simulink model "sensor_fusion"  (R2026a)
settings: Solver=ode1  StopTime=Inf  FixedStep=1/60
PostLoadFcn:
  | qlabs_setup
model workspace (MAT data in the model file):
  lidarStepSize = 0.2
  mainStepSize = Simulink.Parameter
  mainStepSize.Value = Simulink.data.Expression
  mainStepSize.Value.ExpressionString = "qc_get_step_size"
  mainStepSize.Complexity = 'real'
  mainStepSize.Dimensions = -1
  mainStepSize.DataType = 'auto'
  mode = Simulink.Parameter
  mode.Value = 1
  mode.Complexity = 'real'
  mode.Dimensions = [1 1]
  mode.Description = '0 - education speeds via wheel speed commands
    | 1 - education speeds via body speed commands
    | 2 - research speeds via wheel speed commands
    | 3 - research speeds via body speed commands'
  mode.DataType = 'auto'
  realSenseStepSize = Simulink.Parameter
  realSenseStepSize.Value = Simulink.data.Expression
  realSenseStepSize.Value.ExpressionString = "qc_get_step_size*ceil(1/30/qc_get_step_size)"
  realSenseStepSize.Complexity = 'real'
  realSenseStepSize.Dimensions = -1
  realSenseStepSize.DataType = 'auto'
undefined symbols (not defined in the file or in its folder): Point
libraries: quarc_library x17, simulink x1
settings Model: ExtModeTrigDuration=10000  Creator=mbohra  LastModifiedBy=rdu
settings DebuggingCC: UnderspecifiedInitializationDetection=Classic
settings SimscapeCC: SimscapeNominalValues="[{\"value\":\"1\",\"unit\":\"A\"},{\"value\":\"1\",\"unit\":\"bar\"},{\"value\":\"1\",\"unit\":\"cm^2\"},{\"value\":\"1\",\"unit\":\"cm^3/s\"},{\"value\":\"1\",\"unit\":\"kJ/kg\"},{\"value\":\"1\",\"unit\":\"kW\"},{\"value\":\"1\",\"unit\":\"l\"},{\"value\":\"1\",\"unit\":\"N\"},{\"value\":\"1\",\"unit\":\"N*m\"},{\"value\":\"1\",\"unit\":\"V\"}]"  SimscapeLogType=none  SimscapeLogDataHistory=5000.0

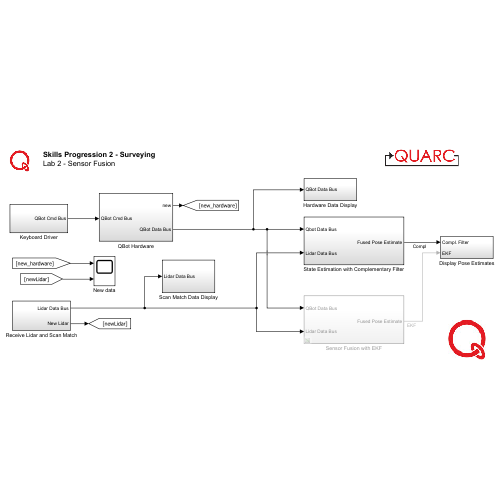
[thumbnail: Simulink's stored preview of the top-level diagram]
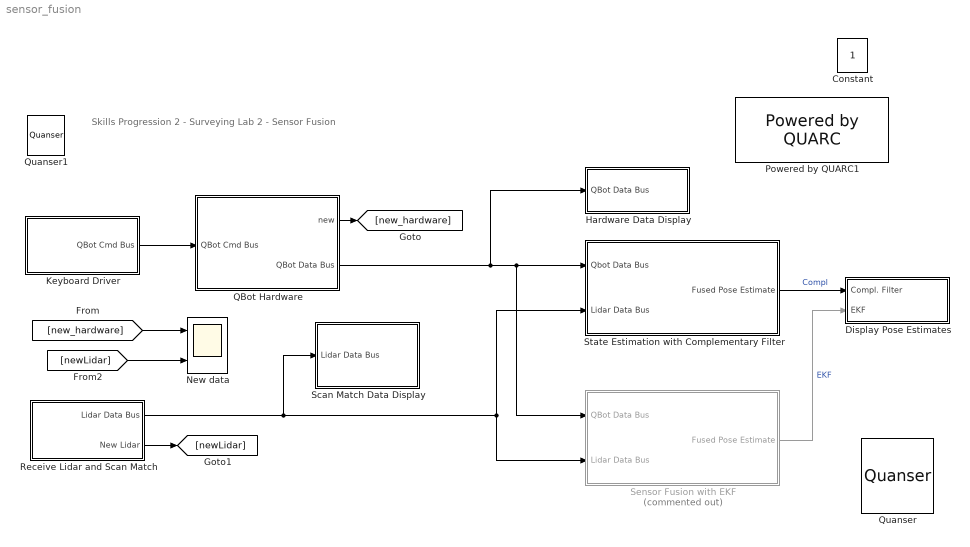
== system sensor_fusion ==
  note: Skills Progression 2 - Surveying
      | Lab 2 - Sensor Fusion
  Display Pose Estimates : Subsystem
  Hardware Data Display : Subsystem
  Keyboard Driver : Subsystem
  New data : Scope  NumInputPorts=2
      settings: Title=Lidar Data New?  ActiveDisplayYMinimum=0.91645239282911062  ActiveDisplayYMaximum=1.0809928877874873  DataLoggingVariableName=ScopeData2
  Powered by QUARC1 : quarc_library/Logos/Powered by QUARC
  QBot Hardware : Subsystem
  Quanser : quarc_library/Logos/Quanser
  Quanser1 : quarc_library/Logos/Quanser
  Receive Lidar and Scan Match : Subsystem
  Scan Match Data Display : Subsystem
  Sensor Fusion with EKF : Subsystem  Commented=on
  State Estimation with Complementary Filter : Subsystem
  Constant : Constant  IOType=siggen  VectorParams1D=off  SampleTime=1
  wires:
  QBot Hardware/2(QBot Data Bus) -> State Estimation with Complementary Filter/1(Qbot Data Bus), Sensor Fusion with EKF/1(QBot Data Bus), Hardware Data Display/1(QBot Data Bus)
  QBot Hardware/1(new) -> [new_hardware]
  [newLidar] -> New data/2
  [new_hardware] -> New data/1
  Keyboard Driver/1(QBot Cmd Bus) -> QBot Hardware/1(QBot Cmd Bus)
  Receive Lidar and Scan Match/1(Lidar Data Bus) -> Scan Match Data Display/1(Lidar Data Bus), Sensor Fusion with EKF/2(Lidar Data Bus), State Estimation with Complementary Filter/2(Lidar Data Bus)
  Receive Lidar and Scan Match/2(New Lidar) -> [newLidar]
  State Estimation with Complementary Filter/1(Fused Pose Estimate) -> Display Pose Estimates/1(Compl. Filter)  "Compl"
  Sensor Fusion with EKF/1(Fused Pose Estimate) -> Display Pose Estimates/2(EKF)  "EKF"

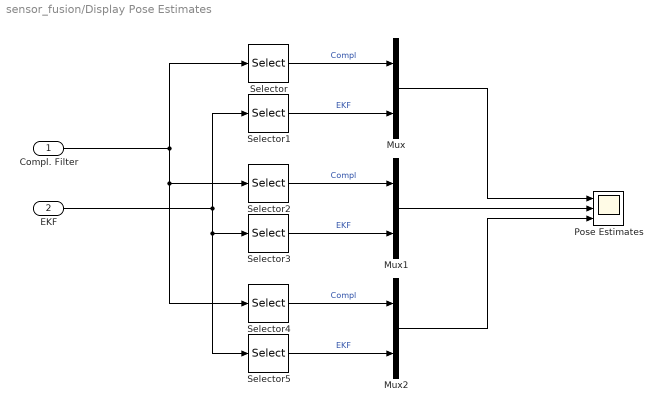
== system sensor_fusion/Display Pose Estimates ==
  Compl. Filter : Inport
  EKF : Inport  Port=2
  Mux : Mux  Inputs=2
  Mux1 : Mux  Inputs=2
  Mux2 : Mux  Inputs=2
  "Pose Estimates " : Scope  NumInputPorts=3
      settings: ActiveDisplayString=3  Title=Theta (rad)  ActiveDisplayYMinimum=-3.7845885644041823  ActiveDisplayYMaximum=8.5346333601811839  DataLoggingVariableName=ScopeData4
  Selector : Selector  InputPortWidth=3  IndexOptions=Index vector (dialog)  Indices=[1]  OutputSizes=1
  Selector1 : Selector  InputPortWidth=3  IndexOptions=Index vector (dialog)  Indices=[1]  OutputSizes=1
  Selector2 : Selector  InputPortWidth=3  IndexOptions=Index vector (dialog)  Indices=[2]  OutputSizes=1
  Selector3 : Selector  InputPortWidth=3  IndexOptions=Index vector (dialog)  Indices=[2]  OutputSizes=1
  Selector4 : Selector  InputPortWidth=3  IndexOptions=Index vector (dialog)  Indices=[3]  OutputSizes=1
  Selector5 : Selector  InputPortWidth=3  IndexOptions=Index vector (dialog)  Indices=[3]  OutputSizes=1
  wires:
  Compl. Filter/1 -> Selector4/1, Selector2/1, Selector/1
  Mux/1 -> "Pose Estimates "/1
  Selector/1 -> Mux/1  "Compl"
  EKF/1 -> Selector5/1, Selector3/1, Selector1/1
  Selector1/1 -> Mux/2  "EKF"
  Selector2/1 -> Mux1/1  "Compl"
  Selector3/1 -> Mux1/2  "EKF"
  Selector5/1 -> Mux2/2  "EKF"
  Selector4/1 -> Mux2/1  "Compl"
  Mux1/1 -> "Pose Estimates "/2
  Mux2/1 -> "Pose Estimates "/3

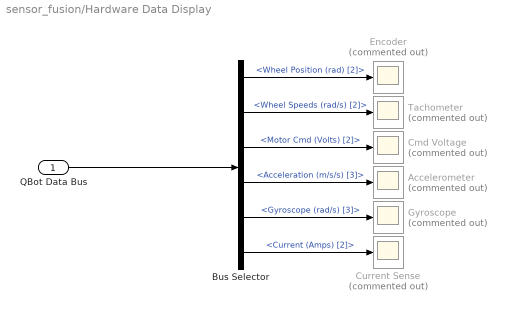
== system sensor_fusion/Hardware Data Display ==
  QBot Data Bus : Inport
  Accelerometer : Scope  Commented=on
      settings: ActiveDisplayYMinimum=-1.32758  ActiveDisplayYMaximum=11.23  DataLoggingVariableName=ScopeData5
  Bus Selector : BusSelector  OutputSignals=Wheel Position (rad) [2],Wheel Speeds (rad/s) [2],Motor Cmd (Volts) [2],Acceleration (m/s/s) [3],Gyroscope (rad/s) [3],Current (Amps) [2]
  Cmd Voltage : Scope  Commented=on
      settings: ActiveDisplayYMinimum=-1  ActiveDisplayYMaximum=1  DataLoggingVariableName=ScopeData4
  Current Sense : Scope  Commented=on
      settings: ActiveDisplayYMinimum=-0.05029  ActiveDisplayYMaximum=0.45265  DataLoggingVariableName=ScopeData7
  Encoder : Scope  Commented=on
      settings: ActiveDisplayYMinimum=-23.46955  ActiveDisplayYMaximum=23.65434  DataLoggingVariableName=ScopeData8
  Gyroscope : Scope  Commented=on
      settings: ActiveDisplayYMinimum=-0.40322  ActiveDisplayYMaximum=1.99912  DataLoggingVariableName=ScopeData6
  Tachometer : Scope  Commented=on
      settings: ActiveDisplayYMinimum=-11.69986  ActiveDisplayYMaximum=11.67552  DataLoggingVariableName=ScopeData3
  wires:
  Bus Selector/2 -> Tachometer/1  "<Wheel Speeds (rad/s) [2]>"
  Bus Selector/6 -> Current Sense/1  "<Current (Amps) [2]>"
  Bus Selector/3 -> Cmd Voltage/1  "<Motor Cmd (Volts) [2]>"
  Bus Selector/4 -> Accelerometer/1  "<Acceleration (m/s/s) [3]>"
  Bus Selector/5 -> Gyroscope/1  "<Gyroscope (rad/s) [3]>"
  Bus Selector/1 -> Encoder/1  "<Wheel Position (rad) [2]>"
  QBot Data Bus/1 -> Bus Selector/1

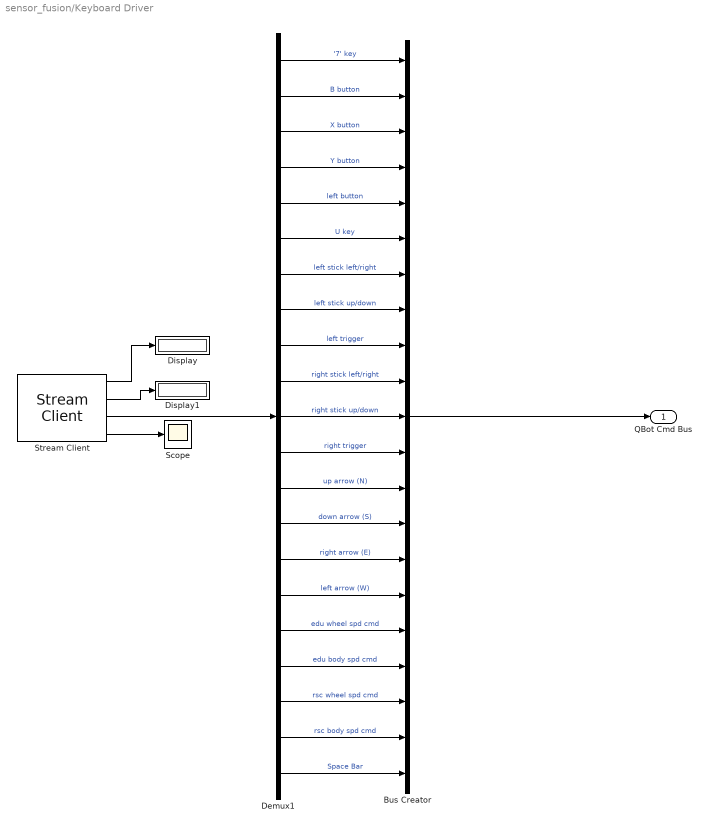
== system sensor_fusion/Keyboard Driver ==
  Bus Creator : BusCreator  Inputs=21
  Demux1 : Demux  Outputs=[1 1 1 1 1 1 1 1 1 1 1 1 1 1 1 1 2 2 2 2 1]
  Display : Display
  Display1 : Display
  Scope : Scope
      settings: ActiveDisplayYMinimum=-0.125  ActiveDisplayYMaximum=1.125
  Stream Client : quarc_library/Communications/Basic/Stream Client  uri_source=Specify via dialog (do not evaluate)  uri=tcpip://localhost:18889?nagle='off'  send_buffer_size=1460  receive_buffer_size=1460  byte_order=little endian (Intel - LSB first)  optimization=Minimum latency  send_options=Do not send data  receive_options=Receive most recent data  default_value=zeros(25,1)  sample_time=mainStepSize  active=on  implementation=Use blocking I/O in a separate thread  send_fifo_size=1000  receive_fifo_size=1000  send_priority=0  receive_priority=0  send_dimensions=off  receive_dimensions=off  max_dimensions=-1  data_type=Inherited via back propagation  type_expr=BusObject
      settings: AttributesFormatString="\"tcpip://localhost:18889?nagle='off'\""
  QBot Cmd Bus : Outport
  wires:
  Bus Creator/1 -> QBot Cmd Bus/1
  Stream Client/3 -> Demux1/1
  Demux1/1 -> Bus Creator/1  "'7' key"
  Demux1/2 -> Bus Creator/2  "B button"
  Demux1/3 -> Bus Creator/3  "X button"
  Demux1/4 -> Bus Creator/4  "Y button"
  Demux1/5 -> Bus Creator/5  "left button"
  Demux1/6 -> Bus Creator/6  "U key"
  Demux1/7 -> Bus Creator/7  "left stick left/right"
  Demux1/8 -> Bus Creator/8  "left stick up/down"
  Demux1/9 -> Bus Creator/9  "left trigger"
  Demux1/10 -> Bus Creator/10  "right stick left/right"
  Demux1/11 -> Bus Creator/11  "right stick up/down"
  Demux1/12 -> Bus Creator/12  "right trigger"
  Demux1/13 -> Bus Creator/13  "up arrow (N)"
  Demux1/14 -> Bus Creator/14  "down arrow (S)"
  Demux1/15 -> Bus Creator/15  "right arrow (E)"
  Demux1/16 -> Bus Creator/16  "left arrow (W)"
  Demux1/17 -> Bus Creator/17  "edu wheel spd cmd"
  Demux1/18 -> Bus Creator/18  "edu body spd cmd"
  Demux1/19 -> Bus Creator/19  "rsc wheel spd cmd"
  Demux1/20 -> Bus Creator/20  "rsc body spd cmd"
  Demux1/21 -> Bus Creator/21  "Space Bar"
  Stream Client/1 -> Display/1
  Stream Client/2 -> Display1/1
  Stream Client/4 -> Scope/1

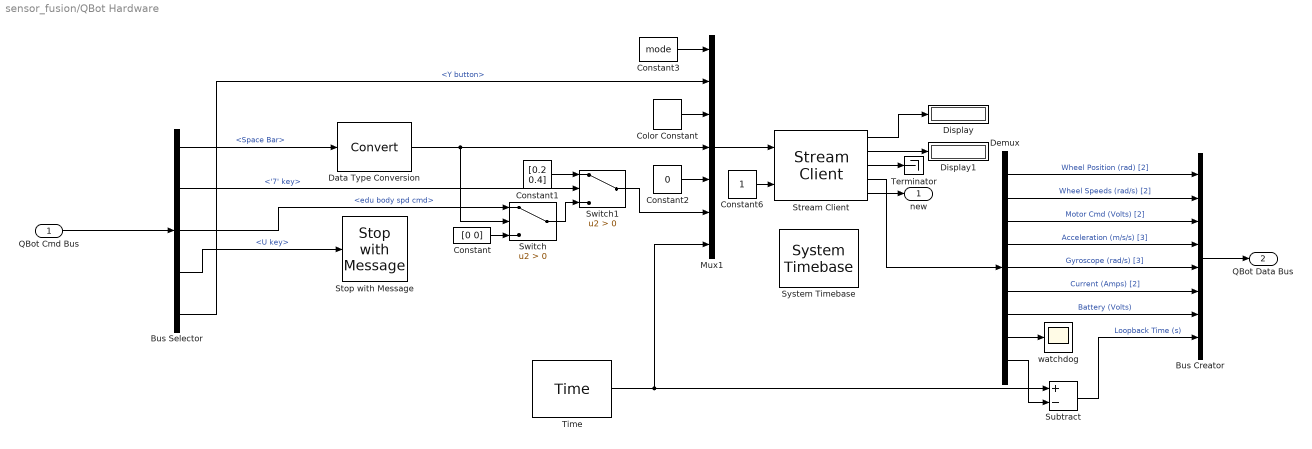
== system sensor_fusion/QBot Hardware ==
  QBot Cmd Bus : Inport
  Bus Creator : BusCreator  Inputs=8
  Bus Selector : BusSelector  OutputSignals=Space Bar,'7' key,edu body spd cmd,U key,Y button
  Color Constant : quarc_library/Sources/Signals/Color Constant  color=[1 0 1]
      settings: SourceProductName=QUARC Targets
  Constant : Constant  Value=[0 0]
  Constant1 : Constant  Value=[0.2 0.4]
  Constant2 : Constant  Value=0
  Constant3 : Constant  Value=mode
  Constant6 : Constant
  Data Type Conversion : DataTypeConversion  SaturateOnIntegerOverflow=off  RndMeth=Floor
  Demux : Demux  Outputs=[2 2 2 3 3 2 1 1 1]
  Display : Display
  Display1 : Display
  Mux1 : Mux  Inputs=7
  Stop with Message : quarc_library/Sinks/Error Handling/Stop with Message  message_type=Fixed error message  message_icon=Information  message=Operator: Emergency Stop
  Stream Client : quarc_library/Communications/Basic/Stream Client  uri_source=Specify via dialog (do not evaluate)  uri=tcpip://localhost:18888  send_buffer_size=1460  receive_buffer_size=1460  byte_order=little endian (Intel - LSB first)  optimization=Minimum latency  send_options=Send most recent data  receive_options=Receive most recent data  default_value=zeros(17,1)  sample_time=mainStepSize  active=on  implementation=Use blocking I/O in a separate thread  send_fifo_size=1000  receive_fifo_size=1000  send_priority=0  receive_priority=0  send_dimensions=off  receive_dimensions=off  max_dimensions=-1  data_type=Inherited via back propagation  type_expr=BusObject
      settings: AttributesFormatString="\"tcpip://localhost:18888\""
  Subtract : Sum  Inputs=+-
  Switch : Switch  Criteria=u2 > Threshold  SaturateOnIntegerOverflow=off  InputSameDT=off
  Switch1 : Switch  Criteria=u2 > Threshold  SaturateOnIntegerOverflow=off  InputSameDT=off
  System Timebase : quarc_library/Advanced/Timing/System Timebase  stop_on_overrun=off
      settings: SourceProductName=QUARC Targets
  Terminator : Terminator
  Time : quarc_library/Sources/Time/Time  time_source=Wall clock  sample_time=qc_get_step_size
  watchdog : Scope
  new : Outport
  QBot Data Bus : Outport  Port=2
  wires:
  Demux/2 -> Bus Creator/2  "Wheel Speeds (rad/s) [2]"
  Constant3/1 -> Mux1/1
  Stream Client/3 -> Terminator/1
  Bus Selector/3 -> Switch/1  "<edu body spd cmd>"
  Stream Client/1 -> Display/1
  Constant6/1 -> Stream Client/2
  Stream Client/2 -> Display1/1
  Color Constant/1 -> Mux1/3
  Demux/3 -> Bus Creator/3  "Motor Cmd (Volts) [2]"
  Mux1/1 -> Stream Client/1
  Stream Client/4 -> Demux/1
  Demux/1 -> Bus Creator/1  "Wheel Position (rad) [2]"
  Stream Client/5 -> new/1
  Demux/7 -> Bus Creator/7  "Battery (Volts)"
  Demux/5 -> Bus Creator/5  "Gyroscope (rad/s) [3]"
  Demux/6 -> Bus Creator/6  "Current (Amps) [2]"
  Demux/9 -> Subtract/2
  Constant2/1 -> Mux1/5
  Demux/4 -> Bus Creator/4  "Acceleration (m/s/s) [3]"
  Time/1 -> Mux1/7, Subtract/1
  Bus Creator/1 -> QBot Data Bus/1
  Subtract/1 -> Bus Creator/8  "Loopback Time (s)"
  Demux/8 -> watchdog/1
  Constant/1 -> Switch/3
  QBot Cmd Bus/1 -> Bus Selector/1
  Bus Selector/4 -> Stop with Message/1  "<U key>"
  Bus Selector/1 -> Data Type Conversion/1  "<Space Bar>"
  Bus Selector/5 -> Mux1/2  "<Y button>"
  Data Type Conversion/1 -> Mux1/4, Switch/2
  Bus Selector/2 -> Switch1/2  "<'7' key>"
  Switch1/1 -> Mux1/6
  Switch/1 -> Switch1/3
  Constant1/1 -> Switch1/1

== system sensor_fusion/Receive Lidar and Scan Match ==
  Bus Creator : BusCreator  Inputs=5
  Demux1 : Demux  Outputs=[210 210 1 1 1]
  Display : Display
  Display1 : Display
  Stream Client : quarc_library/Communications/Basic/Stream Client  uri_source=Specify via dialog (do not evaluate)  uri=tcpip://localhost:18001  send_buffer_size=(210*2+3)*8*2  receive_buffer_size=(210*2+3)*8*2  byte_order=little endian (Intel - LSB first)  optimization=Minimum latency  send_options=Do not send data  receive_options=Receive most recent data  default_value=zeros(423,1)  sample_time=qc_get_step_size  active=on  implementation=Use non-blocking I/O  send_fifo_size=1000  receive_fifo_size=2  send_priority=0  receive_priority=0  send_dimensions=off  receive_dimensions=off  max_dimensions=-1  data_type=Inherited via back propagation  type_expr=BusObject
      settings: AttributesFormatString="\"tcpip://localhost:18001\""
  Lidar Data Bus : Outport
  New Lidar : Outport  Port=2
  wires:
  Stream Client/4 -> New Lidar/1
  Stream Client/1 -> Display1/1
  Stream Client/2 -> Display/1
  Stream Client/3 -> Demux1/1
  Demux1/1 -> Bus Creator/1  "reference ranges"
  Demux1/2 -> Bus Creator/2  "reference angles"
  Demux1/3 -> Bus Creator/3  "x"
  Demux1/4 -> Bus Creator/4  "y"
  Demux1/5 -> Bus Creator/5  "theta"
  Bus Creator/1 -> Lidar Data Bus/1

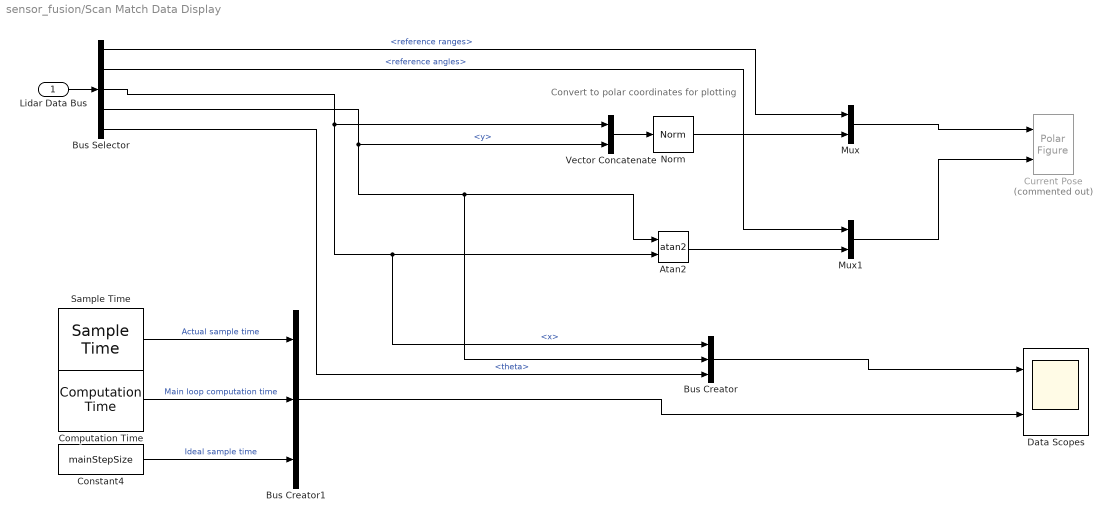
== system sensor_fusion/Scan Match Data Display ==
  note: Convert to polar coordinates for plotting
  Lidar Data Bus : Inport
  Atan2 : Trigonometry  Operator=atan2
  Bus Creator : BusCreator  Inputs=3
  Bus Creator1 : BusCreator  Inputs=3
  Bus Selector : BusSelector  OutputSignals=reference ranges,reference angles,x,y,theta
  Computation Time : quarc_library/Sources/Time/Computation Time  sample_time=qc_get_step_size  use_model=on  use_cpu_time=off
  Constant4 : Constant  Value=mainStepSize
  Current Pose : quarc_library/Sinks/Figures/Polar Figure  Commented=on  figure_mode=Use figure window  figure_tag=figure1  axes_tag=axes1  plot_mode=Frame-based  minimum_rho=0  maximum_rho=2  minimum_theta=0  maximum_theta=360  zero_location=right  direction=counterclockwise  buffer_size=2  update_rate=1  sample_time=-1  initial_position="3218   316   471   457"  initial_visibility=off  line1_style=None  line1_width=0.5  line1_color=[1 0 0]  marker1=Point (.)  marker1_size=6  marker1_edge_color=[1 0 0]  marker1_face_color=[1 0 0]  line2_style=Solid line (-)  line2_width=0.5  line2_color=[0.85098 0.32549 0.0980392]  marker2=None  marker2_size=6  marker2_edge_color=[0.85098 0.32549 0.0980392]  marker2_face_color=[0.85098 0.32549 0.0980392]  line3_style=Solid line (-)  line3_width=0.5  line3_color=[0.929412 0.694118 0.12549]  marker3=None  marker3_size=6  marker3_edge_color=[0.929412 0.694118 0.12549]  marker3_face_color=[0.929412 0.694118 0.12549]  line4_style=Solid line (-)  line4_width=0.5  line4_color=[0.494118 0.184314 0.556863]  marker4=None  marker4_size=6  marker4_edge_color=[0.494118 0.184314 0.556863]  marker4_face_color=[0.494118 0.184314 0.556863]  line5_style=Solid line (-)  line5_width=0.5  line5_color=[0.466667 0.67451 0.188235]  marker5=None  marker5_size=6  marker5_edge_color=[0.466667 0.67451 0.188235]  marker5_face_color=[0.466667 0.67451 0.188235]
      settings: SourceProductName=QUARC Targets
  Data Scopes : Scope  NumInputPorts=2
      settings: Title=Timing  ActiveDisplayYMinimum=-0.0093233205491243983  ActiveDisplayYMaximum=0.025642946758140522
  Mux : Mux  Inputs=2
  Mux1 : Mux  Inputs=2
  Norm : quarc_library/Math Operations/Vectors/Norm
      settings: SourceProductName=QUARC Targets
  Sample Time : quarc_library/Sources/Time/Sample Time  Priority=-99  sample_time=qc_get_step_size
  Vector Concatenate : Concatenate
  wires:
  Bus Selector/5 -> Bus Creator/3  "<theta>"
  Bus Selector/3 -> Bus Creator/1, Atan2/2, Vector Concatenate/1  "<x>"
  Bus Selector/4 -> Bus Creator/2, Atan2/1, Vector Concatenate/2  "<y>"
  Bus Creator/1 -> Data Scopes/1
  Sample Time/1 -> Bus Creator1/1  "Actual sample time"
  Computation Time/1 -> Bus Creator1/2  "Main loop computation time"
  Constant4/1 -> Bus Creator1/3  "Ideal sample time"
  Atan2/1 -> Mux1/2
  Norm/1 -> Mux/2
  Vector Concatenate/1 -> Norm/1
  Mux/1 -> Current Pose/1
  Mux1/1 -> Current Pose/2
  Bus Creator1/1 -> Data Scopes/2
  Lidar Data Bus/1 -> Bus Selector/1
  Bus Selector/1 -> Mux/1  "<reference ranges>"
  Bus Selector/2 -> Mux1/1  "<reference angles>"

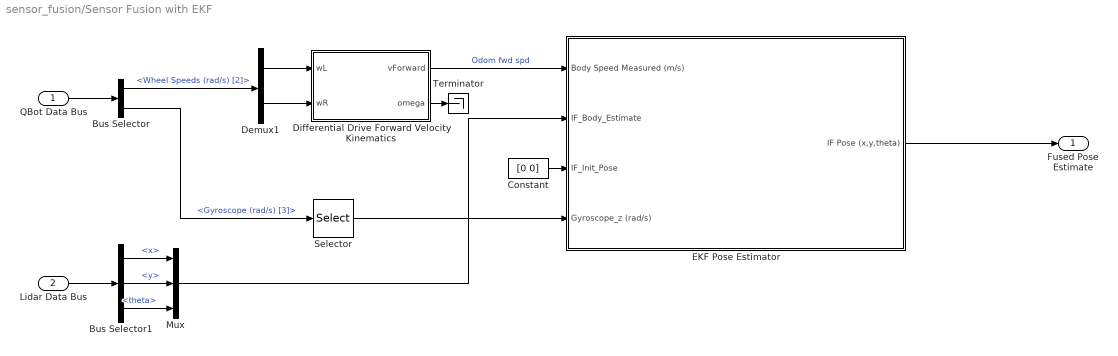
== system sensor_fusion/Sensor Fusion with EKF ==
  QBot Data Bus : Inport
  Lidar Data Bus : Inport  Port=2
  Bus Selector : BusSelector  OutputSignals=Wheel Speeds (rad/s) [2],Gyroscope (rad/s) [3]
  Bus Selector1 : BusSelector  OutputSignals=x,y,theta
  Constant : Constant  Value=[0 0]
  Demux1 : Demux  Outputs=2
  Differential Drive Forward Velocity Kinematics : MATLAB Function  TreatAsAtomicUnit=on
  EKF Pose Estimator : Subsystem
  Mux : Mux  Inputs=3
  Selector : Selector  InputPortWidth=3  IndexOptions=Index vector (dialog)  Indices=[3]  OutputSizes=1
  Terminator : Terminator
  Fused Pose Estimate : Outport
  wires:
  QBot Data Bus/1 -> Bus Selector/1
  Demux1/1 -> Differential Drive Forward Velocity Kinematics/1(wL)
  Demux1/2 -> Differential Drive Forward Velocity Kinematics/2(wR)
  Bus Selector/1 -> Demux1/1  "<Wheel Speeds (rad/s) [2]>"
  Differential Drive Forward Velocity Kinematics/1(vForward) -> EKF Pose Estimator/1(Body Speed Measured (m/s))  "Odom fwd spd"
  Bus Selector/2 -> Selector/1  "<Gyroscope (rad/s) [3]>"
  Selector/1 -> EKF Pose Estimator/4(Gyroscope_z (rad/s))
  EKF Pose Estimator/1(IF Pose (x,y,theta)) -> Fused Pose Estimate/1
  Constant/1 -> EKF Pose Estimator/3(IF_Init_Pose)
  Differential Drive Forward Velocity Kinematics/2(omega) -> Terminator/1
  Lidar Data Bus/1 -> Bus Selector1/1
  Bus Selector1/1 -> Mux/1  "<x>"
  Bus Selector1/2 -> Mux/2  "<y>"
  Bus Selector1/3 -> Mux/3  "<theta>"
  Mux/1 -> EKF Pose Estimator/2(IF_Body_Estimate)

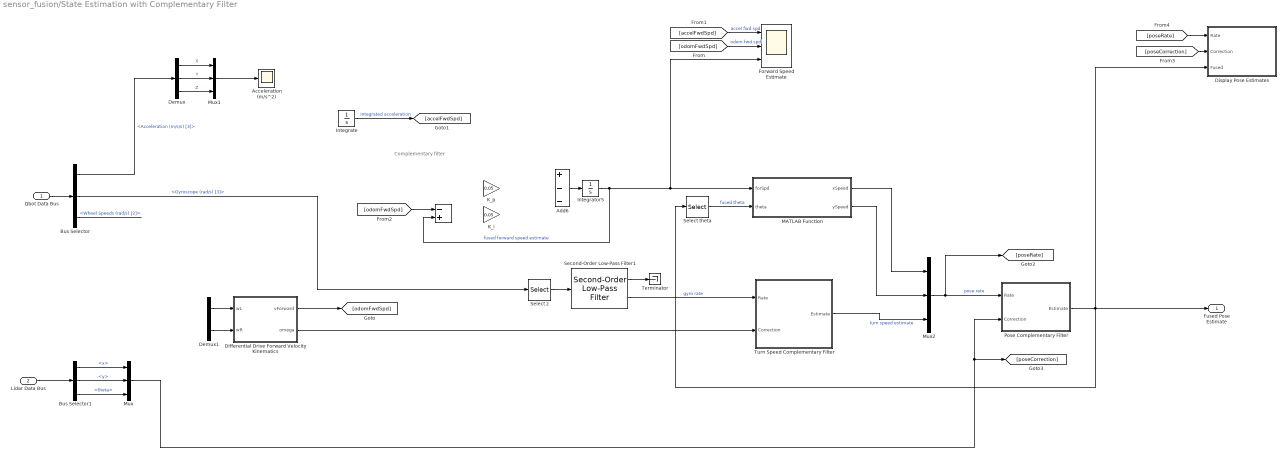
== system sensor_fusion/State Estimation with Complementary Filter ==
  note: Complementary filter
  Qbot Data Bus : Inport
  Lidar Data Bus : Inport  Port=2
  " " : Sum  Inputs=-+
  Acceleration (m/s^2) : Scope
      settings: TimeSpan=10  ActiveDisplayYMinimum=-0.21830889279586507  ActiveDisplayYMaximum=0.25440172069065836  DataLoggingVariableName=ScopeData10
  Add6 : Sum  Inputs=+--
  Bus Selector : BusSelector  OutputSignals=Acceleration (m/s/s) [3],Gyroscope (rad/s) [3],Wheel Speeds (rad/s) [2]
  Bus Selector1 : BusSelector  OutputSignals=x,y,theta
  Demux : Demux  Outputs=3
  Demux1 : Demux  Outputs=2
  Differential Drive Forward Velocity Kinematics : MATLAB Function  TreatAsAtomicUnit=on
  Display Pose Estimates : Subsystem
  Forward Speed Estimate : Scope  NumInputPorts=3
      settings: TimeSpan=10  Title=Forward Speed Estimate  ActiveDisplayYMinimum=-0.27758895946328777  ActiveDisplayYMaximum=0.30244065552015376  DataLoggingVariableName=ScopeData9
  Integrate : Integrator
  Integrator5 : Integrator
  K_i : Gain  Gain=0.05
  K_p : Gain  Gain=0.05
  MATLAB Function : MATLAB Function  TreatAsAtomicUnit=on
  Mux : Mux  Inputs=3
  Mux1 : Mux  Inputs=3
  Mux2 : Mux  Inputs=3
  Pose Complementary Filter : Subsystem
  Second-Order Low-Pass Filter1 : quarc_library/Continuous/Second-Order Low-Pass Filter  params_source=Internal (dialog parameters)  input_width=50  input_zeta=1  input_init=0
  Select theta : Selector  InputPortWidth=3  IndexOptions=Index vector (dialog)  Indices=3  OutputSizes=1
  Select z : Selector  InputPortWidth=3  IndexOptions=Index vector (dialog)  Indices=[3]  OutputSizes=1
  Terminator : Terminator
  Turn Speed Complementary Filter : Subsystem
  Fused Pose Estimate : Outport
  wires:
  Qbot Data Bus/1 -> Bus Selector/1
  Bus Selector/1 -> Demux/1  "<Acceleration (m/s/s) [3]>"
  Demux1/1 -> Differential Drive Forward Velocity Kinematics/1(wL)
  Demux1/2 -> Differential Drive Forward Velocity Kinematics/2(wR)
  Add6/1 -> Integrator5/1
  Demux/2 -> Mux1/2  "Y"
  Demux/3 -> Mux1/3  "Z"
  Mux1/1 -> Acceleration (m/s^2)/1
  [odomFwdSpd] -> Forward Speed Estimate/2  "odom fwd spd"
  [accelFwdSpd] -> Forward Speed Estimate/1  "accel fwd spd"
  Mux2/1 -> [poseRate], Pose Complementary Filter/1(Rate)  "pose rate"
  Integrator5/1 -> MATLAB Function/1(forSpd), Forward Speed Estimate/3, " "/2  "fused forward speed estimate"
  Select theta/1 -> MATLAB Function/2(theta)  "fused theta"
  Second-Order Low-Pass Filter1/2 -> Turn Speed Complementary Filter/1(Rate)  "gyro rate"
  Second-Order Low-Pass Filter1/1 -> Terminator/1
  Integrate/1 -> [accelFwdSpd]  "Integrated acceleration"
  Select z/1 -> Second-Order Low-Pass Filter1/1
  Differential Drive Forward Velocity Kinematics/2(omega) -> Turn Speed Complementary Filter/2(Correction)
  Lidar Data Bus/1 -> Bus Selector1/1
  Bus Selector1/1 -> Mux/1  "<x>"
  Bus Selector1/2 -> Mux/2  "<y>"
  Bus Selector1/3 -> Mux/3  "<theta>"
  Mux/1 -> [poseCorrection], Pose Complementary Filter/2(Correction)
  Bus Selector/2 -> Select z/1  "<Gyroscope (rad/s) [3]>"
  Turn Speed Complementary Filter/1(Estimate) -> Mux2/3  "turn speed estimate"
  Pose Complementary Filter/1(Estimate) -> Display Pose Estimates/3(Fused), Fused Pose Estimate/1, Select theta/1
  MATLAB Function/1(xSpeed) -> Mux2/1
  MATLAB Function/2(ySpeed) -> Mux2/2
  Demux/1 -> Mux1/1  "X"
  Differential Drive Forward Velocity Kinematics/1(vForward) -> [odomFwdSpd]
  [odomFwdSpd] -> " "/1
  [poseRate] -> Display Pose Estimates/1(Rate)
  [poseCorrection] -> Display Pose Estimates/2(Correction)
  ? -> Integrate/1, Add6/1  "fwd accel"
  Bus Selector/3 -> ?  "<Wheel Speeds (rad/s) [2]>"

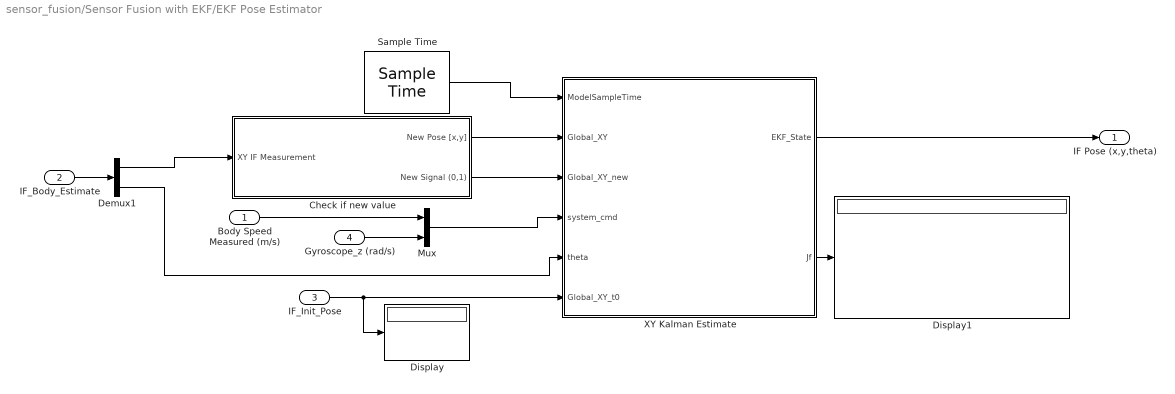
== system sensor_fusion/Sensor Fusion with EKF/EKF Pose Estimator ==
  Body Speed Measured (m/s) : Inport
  IF_Body_Estimate : Inport  Port=2
  IF_Init_Pose : Inport  Port=3
  Gyroscope_z (rad/s) : Inport  Port=4
  Check if new value : Subsystem
  Demux1 : Demux  Outputs=[2,1]
  Display : Display
  Display1 : Display
  Mux : Mux  Inputs=2
  Sample Time : quarc_library/Sources/Time/Sample Time  Priority=-99  sample_time=qc_get_step_size
  XY Kalman Estimate : MATLAB Function  TreatAsAtomicUnit=on
  IF Pose (x,y,theta) : Outport
  wires:
  Sample Time/1 -> XY Kalman Estimate/1(ModelSampleTime)
  Demux1/1 -> Check if new value/1("XY IF Measurement ")
  IF_Init_Pose/1 -> Display/1, XY Kalman Estimate/6(Global_XY_t0)
  IF_Body_Estimate/1 -> Demux1/1
  Check if new value/1(New Pose [x,y]) -> XY Kalman Estimate/2(Global_XY)
  Check if new value/2(New Signal (0,1)) -> XY Kalman Estimate/3(Global_XY_new)
  XY Kalman Estimate/1(EKF_State) -> IF Pose (x,y,theta)/1
  Body Speed Measured (m/s)/1 -> Mux/1
  Mux/1 -> XY Kalman Estimate/4(system_cmd)
  XY Kalman Estimate/2(Jf) -> Display1/1
  Demux1/2 -> XY Kalman Estimate/5(theta)
  Gyroscope_z (rad/s)/1 -> Mux/2

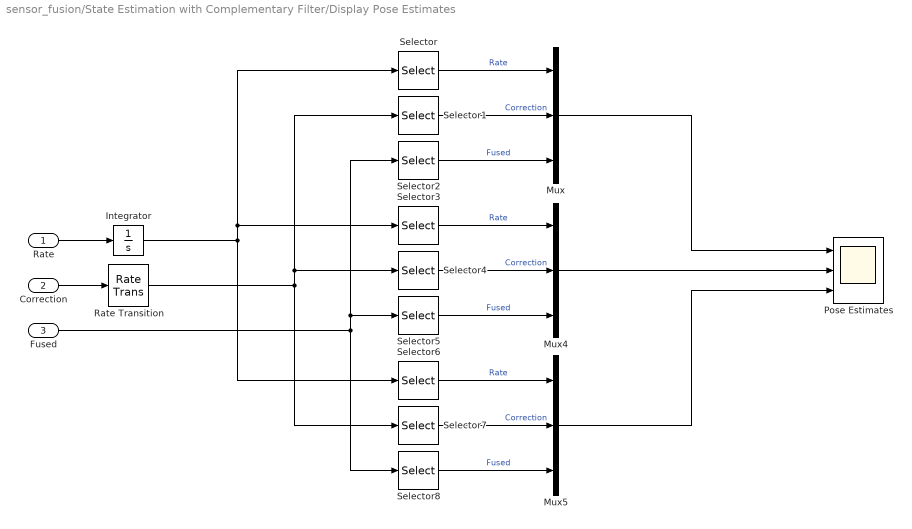
== system sensor_fusion/State Estimation with Complementary Filter/Display Pose Estimates ==
  Rate : Inport
  Correction : Inport  Port=2
  Fused : Inport  Port=3
  Integrator : Integrator
  Mux : Mux  Inputs=3
  Mux4 : Mux  Inputs=3
  Mux5 : Mux  Inputs=3
  Pose Estimates : Scope  NumInputPorts=3
      settings: ActiveDisplayString=3  Title=Theta (rad)  ActiveDisplayYMinimum=-7.2585464207369252  ActiveDisplayYMaximum=7.5280044458771265  DataLoggingVariableName=ScopeData5
  Rate Transition : RateTransition
  Selector : Selector  InputPortWidth=3  IndexOptions=Index vector (dialog)  Indices=[1]  OutputSizes=1
  Selector1 : Selector  InputPortWidth=3  IndexOptions=Index vector (dialog)  Indices=[1]  OutputSizes=1
  Selector2 : Selector  InputPortWidth=3  IndexOptions=Index vector (dialog)  Indices=[1]  OutputSizes=1
  Selector3 : Selector  InputPortWidth=3  IndexOptions=Index vector (dialog)  Indices=[2]  OutputSizes=1
  Selector4 : Selector  InputPortWidth=3  IndexOptions=Index vector (dialog)  Indices=[2]  OutputSizes=1
  Selector5 : Selector  InputPortWidth=3  IndexOptions=Index vector (dialog)  Indices=[2]  OutputSizes=1
  Selector6 : Selector  InputPortWidth=3  IndexOptions=Index vector (dialog)  Indices=[3]  OutputSizes=1
  Selector7 : Selector  InputPortWidth=3  IndexOptions=Index vector (dialog)  Indices=[3]  OutputSizes=1
  Selector8 : Selector  InputPortWidth=3  IndexOptions=Index vector (dialog)  Indices=[3]  OutputSizes=1
  wires:
  Correction/1 -> Rate Transition/1
  Fused/1 -> Selector8/1, Selector5/1, Selector2/1
  Rate Transition/1 -> Selector1/1, Selector4/1, Selector7/1
  Rate/1 -> Integrator/1
  Selector/1 -> Mux/1  "Rate"
  Selector1/1 -> Mux/2  "Correction"
  Selector2/1 -> Mux/3  "Fused"
  Selector3/1 -> Mux4/1  "Rate"
  Selector4/1 -> Mux4/2  "Correction"
  Selector5/1 -> Mux4/3  "Fused"
  Selector6/1 -> Mux5/1  "Rate"
  Selector7/1 -> Mux5/2  "Correction"
  Selector8/1 -> Mux5/3  "Fused"
  Mux/1 -> Pose Estimates/1
  Mux4/1 -> Pose Estimates/2
  Mux5/1 -> Pose Estimates/3
  Integrator/1 -> Selector6/1, Selector/1, Selector3/1

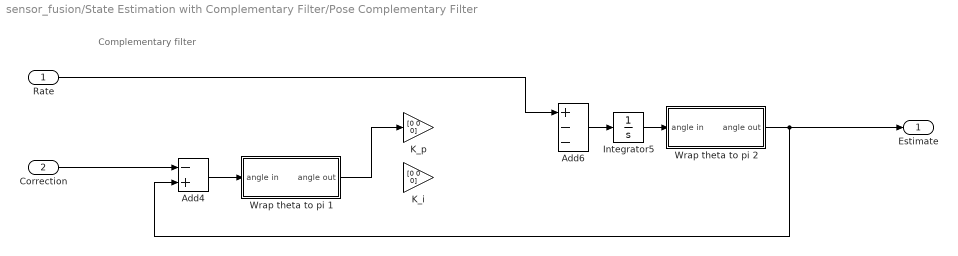
== system sensor_fusion/State Estimation with Complementary Filter/Pose Complementary Filter ==
  note: Complementary filter
  Rate : Inport
  Correction : Inport  Port=2
  Add4 : Sum  Inputs=-+
  Add6 : Sum  Inputs=+--
  Integrator5 : Integrator
  K_i : Gain  Gain=[0 0 0]
  K_p : Gain  Gain=[0 0 0]
  Wrap theta to pi 1 : Subsystem
  Wrap theta to pi 2 : Subsystem
  Estimate : Outport
  wires:
  Add4/1 -> Wrap theta to pi 1/1(angle in)
  Integrator5/1 -> Wrap theta to pi 2/1(angle in)
  Correction/1 -> Add4/1
  Rate/1 -> Add6/1
  Add6/1 -> Integrator5/1
  Wrap theta to pi 2/1(angle out) -> Add4/2, Estimate/1
  Wrap theta to pi 1/1(angle out) -> K_p/1

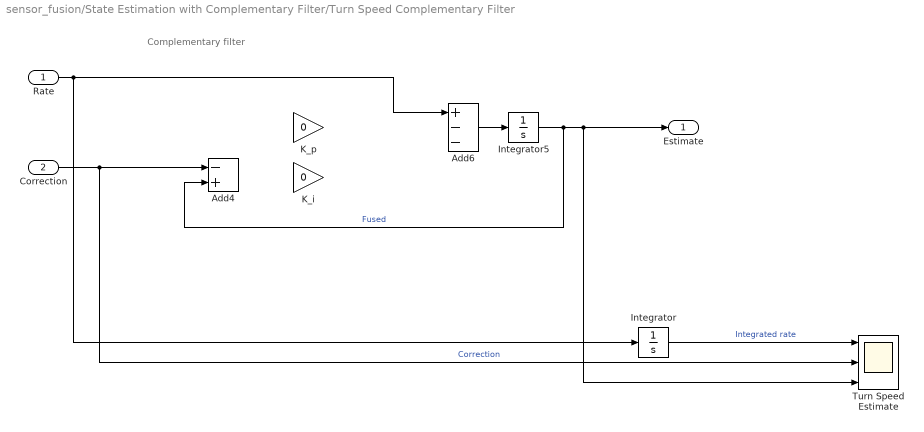
== system sensor_fusion/State Estimation with Complementary Filter/Turn Speed Complementary Filter ==
  note: Complementary filter
  Rate : Inport
  Correction : Inport  Port=2
  Add4 : Sum  Inputs=-+
  Add6 : Sum  Inputs=+--
  Integrator : Integrator
  Integrator5 : Integrator
  K_i : Gain  Gain=0
  K_p : Gain  Gain=0
  Turn Speed Estimate : Scope  NumInputPorts=3
      settings: Title=Turn Speed  ActiveDisplayYMinimum=-0.38759742395959973  ActiveDisplayYMaximum=0.46636210281729384  DataLoggingVariableName=ScopeData11
  Estimate : Outport
  wires:
  Add6/1 -> Integrator5/1
  Rate/1 -> Integrator/1, Add6/1
  Correction/1 -> Turn Speed Estimate/2, Add4/1  "Correction"
  Integrator5/1 -> Turn Speed Estimate/3, Estimate/1, Add4/2  "Fused"
  Integrator/1 -> Turn Speed Estimate/1  "Integrated rate"

== system sensor_fusion/Sensor Fusion with EKF/EKF Pose Estimator/Check if new value ==
  "XY IF Measurement " : Inport
  Detect Change : simulink/Logic and Bit Operations/Detect Change  vinit=0  OutDataTypeStr=boolean
  Memory : Memory
  Norm : quarc_library/Math Operations/Vectors/Norm
      settings: SourceProductName=QUARC Targets
  Switch : Switch  Criteria=u2 > Threshold  SaturateOnIntegerOverflow=off  InputSameDT=off
  New Pose [x,y] : Outport
  New Signal (0,1) : Outport  Port=2
  wires:
  "XY IF Measurement "/1 -> Switch/1, Norm/1
  Norm/1 -> Detect Change/1
  Switch/1 -> New Pose [x,y]/1, Memory/1
  Memory/1 -> Switch/3
  Detect Change/1 -> Switch/2, New Signal (0,1)/1

== system sensor_fusion/State Estimation with Complementary Filter/Pose Complementary Filter/Wrap theta to pi 1 ==
  angle in : Inport
  Assignment : Assignment  DiagnosticForDimensions=Warning  IndexOptions=Index vector (dialog)  Indices=3  OutputSizes=1
  Selector1 : Selector  InputPortWidth=3  IndexOptions=Index vector (dialog)  Indices=[3]  OutputSizes=1
  Wrap theta to pi : MATLAB Function  TreatAsAtomicUnit=on
  angle out : Outport
  wires:
  Assignment/1 -> angle out/1
  Wrap theta to pi/1(y) -> Assignment/2
  Selector1/1 -> Wrap theta to pi/1(u)
  angle in/1 -> Selector1/1, Assignment/1

== system sensor_fusion/State Estimation with Complementary Filter/Pose Complementary Filter/Wrap theta to pi 2 ==
  angle in : Inport
  Assignment : Assignment  DiagnosticForDimensions=Warning  IndexOptions=Index vector (dialog)  Indices=3  OutputSizes=1
  Selector1 : Selector  InputPortWidth=3  IndexOptions=Index vector (dialog)  Indices=[3]  OutputSizes=1
  Wrap theta to pi : MATLAB Function  TreatAsAtomicUnit=on
  angle out : Outport
  wires:
  angle in/1 -> Assignment/1, Selector1/1
  Selector1/1 -> Wrap theta to pi/1(u)
  Wrap theta to pi/1(y) -> Assignment/2
  Assignment/1 -> angle out/1

== matlab function sensor_fusion/Sensor Fusion with EKF/Differential Drive Forward Velocity Kinematics ==
  data: wL input; vForward output; wR input; omega output
function [vForward , omega] = forKin(wL, wR)

% calculate wheel angular velocities
wheelRadius = 3.5*0.0254/2;

vR = wR * wheelRadius;
vL = wL * wheelRadius;

% wheelbase
d=0.3928; 

% calculate wheel linear velocities
vForward = (vR + vL)/2;
omega = (vR - vL)/d;

== matlab function sensor_fusion/State Estimation with Complementary Filter/Pose Complementary Filter/Wrap theta to pi 2/Wrap theta to pi ==
  data: u input; y output
function y = wrap_to_pi(u)
y = atan2(sin(u), cos(u));

== matlab function sensor_fusion/State Estimation with Complementary Filter/Differential Drive Forward Velocity Kinematics ==
  data: wL input; vForward output; wR input; omega output
function [vForward , omega] = forKin(wL, wR)

% calculate wheel angular velocities
wheelRadius = 3.5*0.0254/2;

vR = wR * wheelRadius;
vL = wL * wheelRadius;

% wheelbase
d=0.3928; 

% calculate wheel linear velocities
vForward = (vR + vL)/2;
omega = (vR - vL)/d;

== matlab function sensor_fusion/State Estimation with Complementary Filter/MATLAB Function ==
  data: xSpeed output; ySpeed output; forSpd input; theta input
function [xSpeed,ySpeed] = calculate_xy_speeds(forSpd, theta)
% This function calculates the speeds, in m/s, in the X and Y directions
% using the forward speed, in m/s, and orientation (theta), in rad.

    xSpeed = forSpd*cos(theta);
    ySpeed = forSpd*sin(theta);

end

== matlab function sensor_fusion/State Estimation with Complementary Filter/Pose Complementary Filter/Wrap theta to pi 1/Wrap theta to pi ==
  data: u input; y output
function y = wrap_to_pi(u)
y = atan2(sin(u), cos(u));

== matlab function sensor_fusion/Sensor Fusion with EKF/EKF Pose Estimator/XY Kalman Estimate ==
  data: ModelSampleTime input; Global_XY input; EKF_State output; Global_XY_new input; system_cmd input; theta input; Global_XY_t0 input; Jf output
function [EKF_State, Jf] = fcn( ...
    ModelSampleTime, Global_XY, Global_XY_new, ...
    system_cmd, theta, Global_XY_t0)

%% Extended Kalman Filter for a differential-drive robot
%
% State:
%   x = [X;
%        Y;
%        theta]
%
% Control input:
%   system_cmd(1) = linear velocity  v     [m/s]
%   system_cmd(2) = angular velocity omega [rad/s]
%
% Measurement:
%   Global_XY = measured global position [X,Y]
%   theta     = measured global heading


persistent x P 

%% ---------------------------------------------------------------
% Initialization
% ---------------------------------------------------------------
if isempty(x)

    % Initial EKF state obtained from the initial global pose.
    x = [Global_XY_t0(1);
         Global_XY_t0(2);
         theta];

    % Initial state covariance.
    P = 0.01 * eye(3);

    % First call has no elapsed time.
    dt = 0;

    EKF_State = x;
    Jf = eye(3);

    return;
end

%% ---------------------------------------------------------------
% Calculate elapsed time
% ---------------------------------------------------------------
dt = ModelSampleTime;

% Protection against invalid or zero time steps.
if dt <= 0
    dt = eps;
end

%% ---------------------------------------------------------------
% EKF tuning matrices
% ---------------------------------------------------------------

% Process noise covariance.
%
% These values should eventually be tuned based on the uncertainty in
% the wheel velocity / odometry measurements.
% Q = 0.0075 * eye(3);
Q = diag([0.04 0.04 0.01]);

% Measurement covariance.
%
% Ideally X/Y and theta should have individually tuned variances because
% position is measured in metres while theta is measured in radians.
% R = 0.001 * eye(3);
R = diag([0.005 0.005 1e-4]);

% Full pose measurement matrix:
%
%       z = [X;
%            Y;
%            theta]
%
H = eye(3);

I = eye(3);

%% ---------------------------------------------------------------
% Read control input
% ---------------------------------------------------------------
v     = system_cmd(1);
omega = system_cmd(2);

% IMPORTANT:
% Save heading BEFORE performing the motion prediction.
%
% The Jacobian must be evaluated about the state from which the prediction
% was made, not the already predicted heading.
theta_k = x(3);

%% ===============================================================
% EKF PREDICTION
% ===============================================================

% Threshold used to switch between curved and straight motion models.
omegaThreshold = 0.02;

if abs(omega) > omegaThreshold

    %% -----------------------------------------------------------
    % Exact constant-turn-rate differential-drive motion model
    % -----------------------------------------------------------
    %
    % X(k+1) =
    %   X(k) - v/w*sin(theta)
    %        + v/w*sin(theta + w*dt)
    %
    % Y(k+1) =
    %   Y(k) + v/w*cos(theta)
    %        - v/w*cos(theta + w*dt)
    %
    % theta(k+1) =
    %   theta(k) + w*dt
    %

    theta_next = theta_k + omega*dt;

    x_pred = x + ...
        [-(v/omega)*sin(theta_k) ...
          + (v/omega)*sin(theta_next);

          (v/omega)*cos(theta_k) ...
          - (v/omega)*cos(theta_next);

          omega*dt];

    %% Motion-model Jacobian
    %
    % Jf = df/dx
    Jf = ...
        [1, 0, -(v/omega)*cos(theta_k) ...
                + (v/omega)*cos(theta_next);

         0, 1, -(v/omega)*sin(theta_k) ...
                + (v/omega)*sin(theta_next);

         0, 0, 1];

else

    %% -----------------------------------------------------------
    % Straight-line approximation
    % -----------------------------------------------------------
    %
    % This avoids dividing by omega when omega is approximately zero.
    %

    x_pred = x + ...
        [v*cos(theta_k)*dt;
         v*sin(theta_k)*dt;
         omega*dt];

    %% Straight-motion Jacobian
    Jf = ...
        [1, 0, -v*sin(theta_k)*dt;
         0, 1,  v*cos(theta_k)*dt;
         0, 0,  1];
end

% Normalize predicted heading to [-pi, pi].
x_pred(3) = atan2(sin(x_pred(3)), cos(x_pred(3)));

%% ---------------------------------------------------------------
% Predict covariance
% ---------------------------------------------------------------
P_pred = Jf * P * Jf' + Q;

%% ===============================================================
% EKF MEASUREMENT UPDATE
% ===============================================================

if Global_XY_new

    % Global pose measurement.
    z = [Global_XY(1);
         Global_XY(2);
         theta];

    % Innovation:
    %
    %       innovation = measurement - predicted measurement
    %
    innovation = z - H*x_pred;

    % Heading differences must be normalized.
    %
    % Example:
    %   measured = -179 deg
    %   predicted = +179 deg
    %
    % The error should be +2 deg, not -358 deg.
    innovation(3) = atan2( ...
        sin(innovation(3)), ...
        cos(innovation(3)));

    % Innovation covariance.
    S = H*P_pred*H' + R;

    % Kalman gain.
    %
    % Matrix division is preferred to explicitly computing inv(S).
    K = (P_pred * H') / S;

    % Correct state estimate.
    x = x_pred + K*innovation;

    % Normalize corrected heading.
    x(3) = atan2(sin(x(3)), cos(x(3)));

    % Joseph-form covariance update.
    %
    % This is numerically more robust than:
    %
    %       P = (I-K*H)*P_pred;
    %
    P = (I-K*H)*P_pred*(I-K*H)' + K*R*K';

else

    % No global measurement:
    % prediction becomes the current estimate.
    x = x_pred;
    P = P_pred;
end

%% ---------------------------------------------------------------
% EKF output
% ---------------------------------------------------------------
EKF_State = x;

end
